simulink library "Driver_Long_Lat_Stanley"  (R2020b)
settings: Solver=VariableStepAuto  StartTime=0.0  StopTime=10.0  RelTol=1e-3
undefined symbols (not defined in the file): Driver
libraries: autolibutils x2, simulink x2, autolibsharedcommon x2, drivingvehiclecontroller x1, Maneuver_Get_Pose x1
(part 1 of 2)
Description:
  | Copyright 2020 The MathWorks, Inc.
settings Model: Creator=smiller  LastModifiedBy=smiller
settings DataIOCC: ReturnWorkspaceOutputs=off
settings DebuggingCC: ArithmeticOperatorsInVariantConditions=warning
settings SFSimCC: CustomCodeUndefinedFunction=UseInterfaceOnly

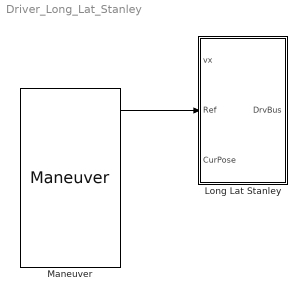
== system Driver_Long_Lat_Stanley ==
  Long Lat Stanley : Subsystem  mask{Driver=Driver}
  Maneuver : Maneuver_Get_Pose/Maneuver  Maneuver=Maneuver  popup_window=No
  wires:
  Maneuver/1 -> Long Lat Stanley/2(Ref)

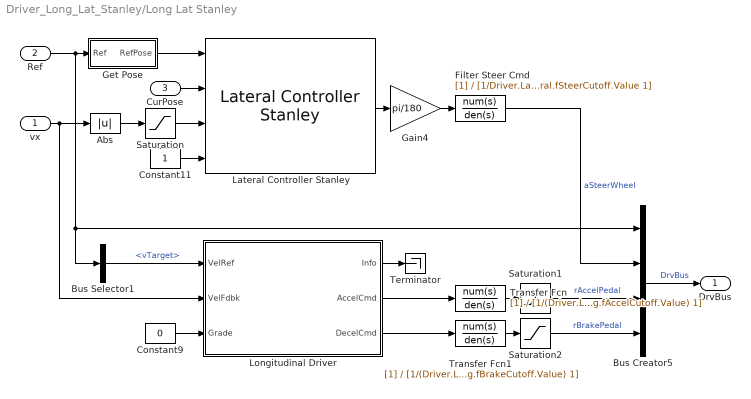
== system Driver_Long_Lat_Stanley/Long Lat Stanley ==
  vx : Inport
  Ref : Inport  Port=2
  CurPose : Inport  Port=3
  Abs : Abs
  Bus Creator5 : BusCreator  Inputs=4
  Bus Selector1 : BusSelector  OutputSignals=vTarget
  Constant11 : Constant
  Constant9 : Constant  Value=0
  Filter Steer Cmd : TransferFcn  Denominator=[1/Driver.Lateral.fSteerCutoff.Value 1]
  Gain4 : Gain  Gain=pi/180
  Get Pose : Subsystem
  Lateral Controller Stanley : drivingvehiclecontroller/Lateral Controller Stanley  ModelType=Kinematic bicycle model  PositionGainF=Driver.Lateral.NForward.Value  PositionGainR=Driver.Lateral.NReverse.Value  YawRateGain=0.2  DelayGain=0.2  VehicleMass=1575  Lf=1.2  Lr=1.6  TireStiffness=19000  Wheelbase=Driver.Lateral.xWheelbase.Value  MaxSteeringAngle=Driver.Lateral.aMaxSteer.Value
      settings: SourceProductName=Automated Driving System Toolbox
  Longitudinal Driver : Subsystem  SystemSampleTime=.01  mask(Longitudinal Driver){extAccelOvr=off, extDecelOvr=off, extAccelHld=off, extDecelHld=off, extAccelZero=off, extDecelZero=off, cntrlType=Predictive, shftType=None, velUnits=m/s, gearOut=off, Kp=15, Ki=1, Kff=.05, Kg=.01, VehVelVec=[0 100], KffVec=[.1 .1], KpVec=[10 10], KiVec=[5 5], KgVec=[0 0], m=Driver.Long.mVehicle.Value, Kpt=Driver.Long.FTractive.Value, tau=Driver.Long.tDriver.Value, L=Driver.Long.xPreview.Value, aR=Driver.Long.NDragRoll.Value, bR=Driver.Long.NDragRollDriveline.Value, cR=Driver.Long.NDragAero.Value, g=Driver.Long.gGravity.Value, vnom=100, Kaw=.1, tauerr=.03, tauPt=2, GearInit=0, tShift=.1, pdlVec=[0.1 0.4 0.5 0.9], upShftTbl=[-1 12.9375 26.4375 39.9375 51.18749999999999 62.4375 72.84375 83.25;-1 16.3125 29.8125 43.3125 54.5624 65.8125 76.78125 87.75;-1 19.6875 33.1875 46.68749999999999 57.9375 69.1875 80.71875 92.25;-1 33 52.5 77.25 100.5 138.75 161.875 185], dwnShftTbl=[1 9.5625 23.0625 36.5625 47.8125 59.0625 68.90625 78.75;1 12.9375 26.4375 39.9375 51.18749999999999 62.4375 72.84375 83.25;1 16.3125 29.8125 43.3125 54.562499 65.8125 76.78125 87.75;1 19.6875 33.1875 46.68749999999999 57.9375 69.1875 80.71875 92.25], tClutch=.5, tRev=.5, tPark=120, aMode=1, UpGearVec=[0  1  2  3  4  5  6  7], DownGearVec=[1  2  3  4  5  6  7  8]}
      mask prompts: extAccelOvr "autoblks_shared:autoblkLongitudinalDriver:blkPrm_extAccelOvr"; extDecelOvr "autoblks_shared:autoblkLongitudinalDriver:blkPrm_extDeccelOvr"; extAccelHld "autoblks_shared:autoblkLongitudinalDriver:blkPrm_extAccelHld"; extDecelHld "autoblks_shared:autoblkLongitudinalDriver:blkPrm_extDeccelHld"; extAccelZero "autoblks_shared:autoblkLongitudinalDriver:blkPrm_extAccelZero"; extDecelZero "autoblks_shared:autoblkLongitudinalDriver:blkPrm_extDeccelZero"; cntrlType "autoblks_shared:autoblkLongitudinalDriver:blkPrm_cntrlType"; shftType "autoblks_shared:autoblkLongitudinalDriver:blkPrm_shftType"; velUnits "autoblks_shared:autoblkLongitudinalDriver:blkPrm_velUnits"; gearOut "autoblks_shared:autoblkLongitudinalDriver:blkPrm_gearOut"; Kp "autoblks_shared:autoblkLongitudinalDriver:blkPrm_Kp"; Ki "autoblks_shared:autoblkLongitudinalDriver:blkPrm_Ki"; Kff "autoblks_shared:autoblkLongitudinalDriver:blkPrm_Kff"; Kg "autoblks_shared:autoblkLongitudinalDriver:blkPrm_Kg"; VehVelVec "autoblks_shared:autoblkLongitudinalDriver:blkPrm_VehVelVec"; KffVec "autoblks_shared:autoblkLongitudinalDriver:blkPrm_KffVec"; KpVec "autoblks_shared:autoblkLongitudinalDriver:blkPrm_KpVec"; KiVec "autoblks_shared:autoblkLongitudinalDriver:blkPrm_KiVec"; KgVec "autoblks_shared:autoblkLongitudinalDriver:blkPrm_KgVec"; m "autoblks_shared:autoblkLongitudinalDriver:blkPrm_m"; Kpt "autoblks_shared:autoblkLongitudinalDriver:blkPrm_Kpt"; tau "autoblks_shared:autoblkLongitudinalDriver:blkPrm_tau"; L "autoblks_shared:autoblkLongitudinalDriver:blkPrm_L"; aR "autoblks_shared:autoblkLongitudinalDriver:blkPrm_aR"; bR "autoblks_shared:autoblkLongitudinalDriver:blkPrm_bR"; cR "autoblks_shared:autoblkLongitudinalDriver:blkPrm_cR"; g "autoblks_shared:autoblkLongitudinalDriver:blkPrm_g"; vnom "autoblks_shared:autoblkLongitudinalDriver:blkPrm_vnom"; Kaw "autoblks_shared:autoblkLongitudinalDriver:blkPrm_Kaw"; tauerr "autoblks_shared:autoblkLongitudinalDriver:blkPrm_tauerr"; tauPt "autoblks_shared:autoblkLongitudinalDriver:blkPrm_tauPt"; GearInit "autoblks_shared:autoblkLongitudinalDriver:blkPrm_GearInit"; tShift "autoblks_shared:autoblkLongitudinalDriver:blkPrm_tShift"; pdlVec "autoblks_shared:autoblkLongitudinalDriver:blkPrm_pdlVec"; upShftTbl "autoblks_shared:autoblkLongitudinalDriver:blkPrm_upShftTbl"; dwnShftTbl "autoblks_shared:autoblkLongitudinalDriver:blkPrm_dwnShftTbl"; tClutch "autoblks_shared:autoblkLongitudinalDriver:blkPrm_tClutch"; tRev "autoblks_shared:autoblkLongitudinalDriver:blkPrm_tRev"; tPark "autoblks_shared:autoblkLongitudinalDriver:blkPrm_tPark"; UpGearVec "autoblks_shared:autoblkLongitudinalDriver:blkPrm_UpGearVec"; DownGearVec "autoblks_shared:autoblkLongitudinalDriver:blkPrm_DownGearVec"
      mask help: autoblks_shared:autoblkLongitudinalDriver:blkDesc
      mask init:
      | [~]=autosharedicon('autoliboperlong',gcb,0);
      mask Help: eval('autosharedhelp(''pbopmodlong'')');
      mask TypeOptions cntrlType: autoblks_shared:autoblkLongitudinalDriver:blkCmb_cntrlType_c1 | autoblks_shared:autoblkLongitudinalDriver:blkCmb_cntrlType_c2 | autoblks_shared:autoblkLongitudinalDriver:blkCmb_cntrlType_c3
      mask Callback cntrlType: [~]=autosharedicon('autoliboperlong',gcb,1);
      mask TypeOptions shftType: Longitudinal Driver/shftType
      mask Callback shftType: [~]=autosharedicon('autoliboperlong',gcb,1);
      mask TypeOptions velUnits: VelRef/Unit
      mask Callback velUnits: [~]=autosharedicon('autoliboperlong',gcb,1);
      mask DialogControl modeConfig Prompt: autoblks_shared:autoblkLongitudinalDriver:blkDlg_modeConfig
      mask DialogControl sigConfigPanel Prompt: autoblks_shared:autoblkLongitudinalDriver:blkDlg_sigConfigPanel
      mask DialogControl extAccelOvr Prompt: Accelerator override
      mask DialogControl extDecelOvr Prompt: Decelerator override
      mask DialogControl extAccelHld Prompt: Accelerator hold
      mask DialogControl extDecelHld Prompt: Decelerator hold
      mask DialogControl extAccelZero Prompt: Accelerator disable
      mask DialogControl extDecelZero Prompt: Decelerator disable
      mask DialogControl cntrlType Prompt: Control type, cntrlType:
      mask DialogControl shftType Prompt: Shift type, shftType:
      mask DialogControl velUnits Prompt: Reference and feedback units, velUnits [velUnits]:
      mask DialogControl gearOut Prompt: Output gear signal
      mask DialogControl CntrlParamPanel Prompt: autoblks_shared:autoblkLongitudinalDriver:blkDlg_CntrlParamPanel
      mask DialogControl PIParam Prompt: autoblks_shared:autoblkLongitudinalDriver:blkDlg_PIParam
      mask DialogControl Kp Prompt: Proportional gain, Kp []:
      mask DialogControl Ki Prompt: Integral gain, Ki []:
      mask DialogControl Kff Prompt: Velocity feed-forward, Kff []:
      mask DialogControl Kg Prompt: Grade angle feed-forward, Kg [1/deg]:
      mask DialogControl PISchedParam Prompt: autoblks_shared:autoblkLongitudinalDriver:blkDlg_PISchedParam
      mask DialogControl VehVelVec Prompt: Velocity gain breakpoints:
      mask DialogControl KffVec Prompt: Velocity feed-forward gain values, KffVec []:
      mask DialogControl KpVec Prompt: Proportional gain values, KpVec []:
      mask DialogControl KiVec Prompt: Integral gain values, KiVec []:
      mask DialogControl KgVec Prompt: Grade angle feed-forward values, KgVec [1/deg]:
      mask DialogControl PredParam Prompt: autoblks_shared:autoblkLongitudinalDriver:blkDlg_PredParam
      mask DialogControl m Prompt: Vehicle mass, m [kg]:
      mask DialogControl Kpt Prompt: Effective vehicle total tractive force, Kpt [N]:
      mask DialogControl tau Prompt: Driver response time, tau [s]:
      mask DialogControl L Prompt: Preview distance, L [m]:
      mask DialogControl aR Prompt: Rolling resistance coefficient, aR [N]:
      mask DialogControl bR Prompt: Rolling and driveline resistance coefficient, bR [N*s/m]:
      mask DialogControl cR Prompt: Aerodynamic drag coefficient, cR [N*s^2/m^2]:
      mask DialogControl g Prompt: Gravitational constant, g [m/s^2]:
      mask DialogControl vnom Prompt: Nominal speed, vnom [velUnits]:
      mask DialogControl Kaw Prompt: Anti-windup, Kaw []:
      mask DialogControl tauerr Prompt: Error filter time constant, tauerr [s]:
      mask DialogControl tauPt Prompt: Powertrain time constant, tauPt [s]:
      mask DialogControl shiftParamPanel Prompt: autoblks_shared:autoblkLongitudinalDriver:blkDlg_shiftParamPanel
      mask DialogControl GearInit Prompt: Initial gear, GearInit []:
      mask DialogControl tShift Prompt: Time required to shift, tShift [s]:
      mask DialogControl pdlVec Prompt: Up and down shift accelerator pedal positions, pdlVec []:
      mask DialogControl upShftTbl Prompt: Upshift velocity data table, upShftTbl [velUnits]:
      mask DialogControl dwnShftTbl Prompt: Downshift velocity data table, dwnShftTbl [velUnits]:
      mask DialogControl tClutch Prompt: Time required to shift, tClutch [s]:
      mask DialogControl tRev Prompt: Time required to engage reverse from neutral, tRev [s]:
      mask DialogControl tPark Prompt: Time required to engage park from neutral, tPark [s]:
      mask DialogControl UpGearVec Prompt: Upshift gear vector, UpGearVec []:
      mask DialogControl DownGearVec Prompt: Downshift gear vector, DownGearVec []:
      mask Display:
      | try
      |     IconInfo = autosharedicon('autoliboperlong', gcb, 4);
      | 
      |     image(IconInfo.image, IconInfo.position);
      | 
      |     for i = 1:numel(IconInfo.lconn)
      |         port_label('lconn', i, IconInfo.lconn{i})
      |     end
      | 
      |     for j = 1:numel(IconInfo.rconn)
      |         port_label('rconn', j, IconInfo.rconn{j})
      |     end
      | 
      |     for k = 1:numel(IconInfo.input)
      |         port_label('input', k, IconInfo.input{k})
      |     end
      | 
      |     for m = 1:numel(IconInfo.output)
      |         port_label('output', m, IconInfo.output{m})
      |     end
      | catch
      |     fprintf('Longitudinal \n Driver')
      | end
  Saturation : Saturate  UpperLimit=inf  LowerLimit=1e-9  ZeroCross=off
  Saturation1 : Saturate  UpperLimit=1  LowerLimit=0  ZeroCross=off
  Saturation2 : Saturate  UpperLimit=1  LowerLimit=0  ZeroCross=off
  Terminator : Terminator
  Transfer Fcn : TransferFcn  Denominator=[1/(Driver.Long.fAccelCutoff.Value) 1]
  Transfer Fcn1 : TransferFcn  Denominator=[1/(Driver.Long.fBrakeCutoff.Value) 1]
  DrvBus : Outport  VectorParamsAs1DForOutWhenUnconnected=off
  wires:
  Constant9/1 -> Longitudinal Driver/3(Grade)
  Bus Creator5/1 -> DrvBus/1  "DrvBus"
  Bus Selector1/1 -> Longitudinal Driver/1(VelRef)  "<vTarget>"
  Gain4/1 -> Filter Steer Cmd/1
  Lateral Controller Stanley/1 -> Gain4/1
  Longitudinal Driver/1(Info) -> Terminator/1
  Longitudinal Driver/2(AccelCmd) -> Transfer Fcn/1
  CurPose/1 -> Lateral Controller Stanley/2
  Longitudinal Driver/3(DecelCmd) -> Transfer Fcn1/1
  Abs/1 -> Saturation/1
  Transfer Fcn1/1 -> Saturation2/1
  Constant11/1 -> Lateral Controller Stanley/4
  Saturation2/1 -> Bus Creator5/4  "rBrakePedal"
  Saturation1/1 -> Bus Creator5/3  "rAccelPedal"
  Transfer Fcn/1 -> Saturation1/1
  vx/1 -> Longitudinal Driver/2(VelFdbk), Abs/1
  Ref/1 -> Bus Creator5/1, Bus Selector1/1, Get Pose/1(Ref)
  Get Pose/1(RefPose) -> Lateral Controller Stanley/1
  Filter Steer Cmd/1 -> Bus Creator5/2  "aSteerWheel"
  Saturation/1 -> Lateral Controller Stanley/3

== system Driver_Long_Lat_Stanley/Long Lat Stanley/Get Pose ==
  Ref : Inport
  Bus Selector : BusSelector  OutputSignals=x,y,ayaw
  Gain : Gain  Gain=180/pi
  Mux : Mux  Inputs=3
  RefPose : Outport  VectorParamsAs1DForOutWhenUnconnected=off
  wires:
  Bus Selector/1 -> Mux/1  "<x>"
  Ref/1 -> Bus Selector/1
  Mux/1 -> RefPose/1
  Bus Selector/2 -> Mux/2  "<y>"
  Bus Selector/3 -> Gain/1  "<ayaw>"
  Gain/1 -> Mux/3

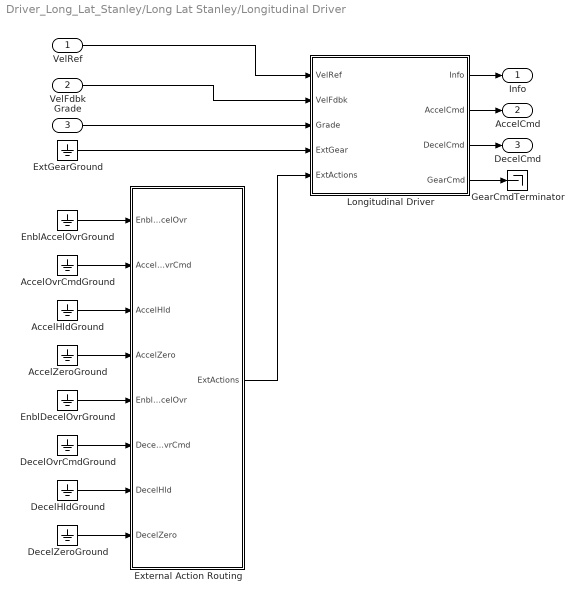
== system Driver_Long_Lat_Stanley/Long Lat Stanley/Longitudinal Driver ==
  VelRef : Inport  Unit=m/s
  VelFdbk : Inport  Port=2  Unit=m/s
  Grade : Inport  Port=3
  AccelHldGround : Ground
  AccelOvrCmdGround : Ground
  AccelZeroGround : Ground
  DecelHldGround : Ground
  DecelOvrCmdGround : Ground
  DecelZeroGround : Ground
  EnblAccelOvrGround : Ground
  EnblDecelOvrGround : Ground
  ExtGearGround : Ground
  External Action Routing : Subsystem
  GearCmdTerminator : Terminator
  Longitudinal Driver : Subsystem  mask(Longitudinal Driver Model){cntrlType=Predictive, shftType=None, vnom=vnom, Kp=Kp, Ki=Ki, Kaw=Kaw, Kff=Kff, Kg=Kg, tauerr=tauerr, tShift=tShift, tRev=tRev, tPark=tPark, pdlVec=pdlVec, upShftTbl=upShftTbl, dwnShftTbl=dwnShftTbl, GearInit=GearInit, tClutch=tClutch, VehVelVec=VehVelVec, KffVec=KffVec, KiVec=KiVec, KpVec=KpVec, KgVec=KgVec, m=m, Kpt=Kpt, Lvv=L, g=g, UpGearVec=UpGearVec, DownGearVec=DownGearVec, aMode=aMode, errUnit=m/s, aR=aR, bR=bR, cR=cR, tauPt=tauPt}
      mask prompts: cntrlType "Control type, cntrlType:"; shftType "Shift type, shftType:"; vnom "Nominal speed, vnom:"; Kp "Proportional gain, Kp:"; Ki "Integral gain, Ki:"; Kaw "Anti-windup, Kaw:"; Kff "Velocity feed-forward, Kff:"; Kg "Grade feed-forward, Kg:"; tauerr "Error filter time constant, tauerr [s]:"; tShift "Time required to shift. tShift [s]:"; tRev "Time required for reverse shift, tRev [s]:"; tPark "Time required to enter park, tPark [s]:"; pdlVec "Up and down shift accelerator pedal positions, pdlVec [-]:"; upShftTbl "Upshift speed data, upShftTbl []:"; dwnShftTbl "Downshift speed data, dwnShftTbl []:"; GearInit "Initial gear, GearInit [-]:"; tClutch "Time requried to shift, tClutch [s]:"; VehVelVec "Velocity gain breakpoints, VehVelVec []:"; KffVec "Velocity feed-forward gain values, KffVec []:Velocity feed-forward gain values, KffVec []:"; KiVec "Integral gain values, KiVec []:"; KpVec "Proportional gain values, KpVec []:"; KgVec "Grade feed-forward values, KgVec []:Grade feed-forward values, KgVec []:Grade feed-forward values, KgVec []:Grade feed-forward values, KgVec []:Grade feed-forward values, KgVec []:"; m "Vehicle mass, m [m]:"; Kpt "Tractive force, Kpt [N]:"; Lvv "Preview distance, Lvv [m]:"; g "Gravitational constant, g, [m/s^2]:"; errUnit "Error units, errUnit"; aR "Static resistance, aR [N]:"; bR "Linear resistance, bR [N*s/m]:"; cR "Quadratic resistance, cR [N*s^2/m^2]:"; tauPt "Powertrain time constant, tauPt [s]:"
      mask help: A parametric longitudinal speed tracking controller for generating normalized acceleration and braking commands based on reference and feedback velocities.
      mask init:
      | [~]=autosharedicon('autoliboperlong',gcb,1);
      mask Help: eval('autoblkshelp(''pbopmodlong'')');
      mask TypeOptions cntrlType: PI | Scheduled PI | Predictive
      mask TypeOptions shftType: None | Reverse, Neutral, Drive | Scheduled | External
      mask TypeOptions errUnit: Routing/error signal spec/Unit
  Info : Outport  InitialOutput=0  VectorParamsAs1DForOutWhenUnconnected=off
  AccelCmd : Outport  Port=2  VectorParamsAs1DForOutWhenUnconnected=off
  DecelCmd : Outport  Port=3  VectorParamsAs1DForOutWhenUnconnected=off
  wires:
  ExtGearGround/1 -> Longitudinal Driver/4(ExtGear)
  Longitudinal Driver/4(GearCmd) -> GearCmdTerminator/1
  EnblDecelOvrGround/1 -> External Action Routing/5(EnblDecelOvr)
  AccelZeroGround/1 -> External Action Routing/4(AccelZero)
  DecelZeroGround/1 -> External Action Routing/8(DecelZero)
  DecelOvrCmdGround/1 -> External Action Routing/6(DecelOvrCmd)
  DecelHldGround/1 -> External Action Routing/7(DecelHld)
  AccelHldGround/1 -> External Action Routing/3(AccelHld)
  EnblAccelOvrGround/1 -> External Action Routing/1(EnblAccelOvr)
  AccelOvrCmdGround/1 -> External Action Routing/2(AccelOvrCmd)
  External Action Routing/1(ExtActions) -> Longitudinal Driver/5(ExtActions)
  Grade/1 -> Longitudinal Driver/3(Grade)
  Longitudinal Driver/3(DecelCmd) -> DecelCmd/1
  Longitudinal Driver/2(AccelCmd) -> AccelCmd/1
  Longitudinal Driver/1(Info) -> Info/1
  VelFdbk/1 -> Longitudinal Driver/2(VelFdbk)
  VelRef/1 -> Longitudinal Driver/1(VelRef)

== system Driver_Long_Lat_Stanley/Long Lat Stanley/Longitudinal Driver/External Action Routing ==
  EnblAccelOvr : Inport  OutDataTypeStr=boolean  Unit=1
  AccelOvrCmd : Inport  Port=2  OutDataTypeStr=double  Unit=1
  AccelHld : Inport  Port=3  OutDataTypeStr=boolean  Unit=1
  AccelZero : Inport  Port=4  OutDataTypeStr=boolean  Unit=1
  EnblDecelOvr : Inport  Port=5  OutDataTypeStr=boolean  Unit=1
  DecelOvrCmd : Inport  Port=6  OutDataTypeStr=double  Unit=1
  DecelHld : Inport  Port=7  OutDataTypeStr=boolean  Unit=1
  DecelZero : Inport  Port=8  OutDataTypeStr=boolean  Unit=1
  Bus Creator2 : BusCreator  Inputs=8
  ExtActions : Outport
  wires:
  Bus Creator2/1 -> ExtActions/1  "ExtActions"
  DecelZero/1 -> Bus Creator2/8  "DecelZero"
  DecelHld/1 -> Bus Creator2/7  "DecelHld"
  DecelOvrCmd/1 -> Bus Creator2/6  "DecelOvrCmd"
  EnblDecelOvr/1 -> Bus Creator2/5  "EnblDecelOvr"
  AccelZero/1 -> Bus Creator2/4  "AccelZero"
  AccelHld/1 -> Bus Creator2/3  "AccelHld"
  AccelOvrCmd/1 -> Bus Creator2/2  "AccelOvrCmd"
  EnblAccelOvr/1 -> Bus Creator2/1  "EnblAccelOvr"

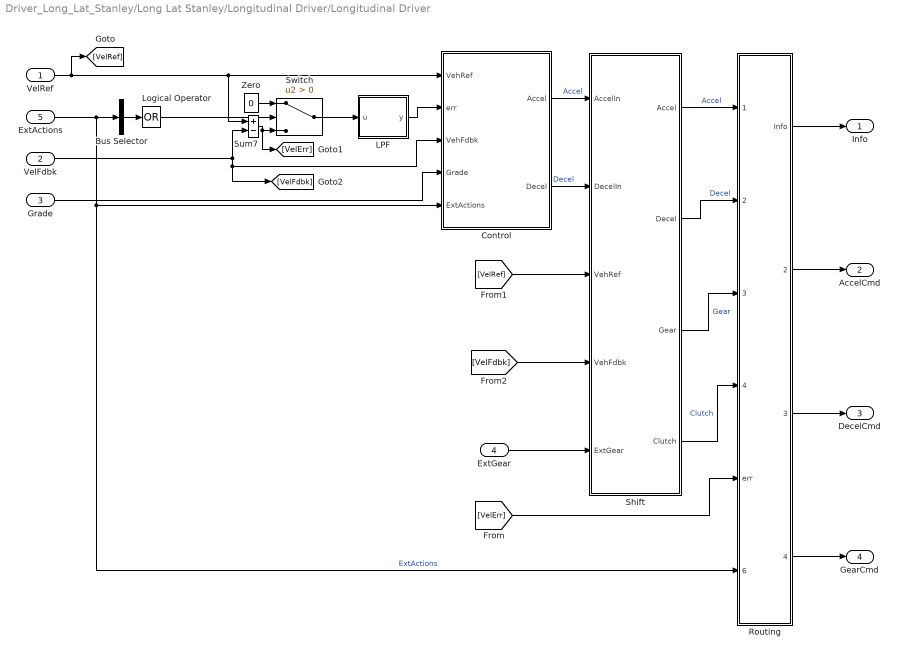
== system Driver_Long_Lat_Stanley/Long Lat Stanley/Longitudinal Driver/Longitudinal Driver ==
  VelRef : Inport
  VelFdbk : Inport  Port=2
  Grade : Inport  Port=3  Unit=deg
  ExtGear : Inport  Port=4  Unit=1
  ExtActions : Inport  Port=5
  Bus Selector : BusSelector  OutputSignals=EnblAccelOvr,AccelHld,AccelZero,EnblDecelOvr,DecelZero,DecelHld  OutputAsBus=on
  Control : Subsystem  Variant=on  VariantControlMode=label  LabelModeActiveChoice=2
  LPF : Subsystem  Variant=on  VariantControlMode=label  LabelModeActiveChoice=0
  Logical Operator : Logic  Operator=OR  Inputs=1  AllPortsSameDT=off  OutDataTypeStr=boolean
  Routing : Subsystem
  Shift : Subsystem  Variant=on  VariantControlMode=label  LabelModeActiveChoice=0
  Sum7 : Sum  Inputs=+-  InputSameDT=on  SaturateOnIntegerOverflow=on  OutDataTypeStr=Inherit: Same as first input
  Switch : Switch  Criteria=u2 > Threshold
  Zero : Constant  Value=0  OutDataTypeStr=Inherit: Inherit via back propagation
  Info : Outport  InitialOutput=0  VectorParamsAs1DForOutWhenUnconnected=off
  AccelCmd : Outport  Port=2  Unit=one  InitialOutput=0  VectorParamsAs1DForOutWhenUnconnected=off
  DecelCmd : Outport  Port=3  Unit=one  InitialOutput=0  VectorParamsAs1DForOutWhenUnconnected=off
  GearCmd : Outport  Port=4  Unit=one  InitialOutput=0  VectorParamsAs1DForOutWhenUnconnected=off
  wires:
  Control/1(Accel) -> Shift/1(AccelIn)  "Accel"
  [VelFdbk] -> Shift/4(VehFdbk)
  Control/2(Decel) -> Shift/2(DecelIn)  "Decel"
  Routing/3(DecelCmd) -> DecelCmd/1
  [VelErr] -> Routing/5(err)
  [VelRef] -> Shift/3(VehRef)
  Routing/4(GearCmd) -> GearCmd/1
  Shift/3(Gear) -> Routing/3(GearIn)  "Gear"
  Routing/1(Info) -> Info/1
  Shift/2(Decel) -> Routing/2(DecelIn)  "Decel"
  Shift/4(Clutch) -> Routing/4(Clutch)  "Clutch"
  Routing/2(AccelCmd) -> AccelCmd/1
  Grade/1 -> Control/4(Grade)
  Sum7/1 -> Switch/3, [VelErr]
  Shift/1(Accel) -> Routing/1(AccelIn)  "Accel"
  LPF/1(y) -> Control/2(err)
  ExtGear/1 -> Shift/5(ExtGear)
  VelRef/1 -> Control/1(VehRef), Sum7/1, [VelRef]
  VelFdbk/1 -> [VelFdbk], Control/3(VehFdbk), Sum7/2
  ExtActions/1 -> Routing/6(ExtActions), Control/5(ExtActions), Bus Selector/1  "ExtActions"
  Switch/1 -> LPF/1(u)
  Logical Operator/1 -> Switch/2
  Zero/1 -> Switch/1
  Bus Selector/1 -> Logical Operator/1

== system Driver_Long_Lat_Stanley/Long Lat Stanley/Longitudinal Driver/Longitudinal Driver/Control ==
  note: 1) Add Subsystem or Model blocks as valid variant choices.
      | 2) You cannot connect blocks at this level. At simulation, connectivity is automatically
      | determined, based on the active variant and port name matching.
  VehRef : Inport
  err : Inport  Port=2
  VehFdbk : Inport  Port=3
  Grade : Inport  Port=4
  ExtActions : Inport  Port=5
  Mapped : Subsystem  VariantControl=1
  Predictive : Subsystem  VariantControl=2
  Scalar : Subsystem  VariantControl=0
  Accel : Outport  VectorParamsAs1DForOutWhenUnconnected=off
  Decel : Outport  Port=2  VectorParamsAs1DForOutWhenUnconnected=off

== system Driver_Long_Lat_Stanley/Long Lat Stanley/Longitudinal Driver/Longitudinal Driver/LPF ==
  note: 1) Add Subsystem or Model blocks as valid variant choices.
      | 2) You cannot connect blocks at this level. At simulation, connectivity is automatically
      | determined, based on the active variant and port name matching.
  u : Inport
  LPF : Subsystem  VariantControl=1
  pass : Subsystem  VariantControl=0
  y : Outport  VectorParamsAs1DForOutWhenUnconnected=off

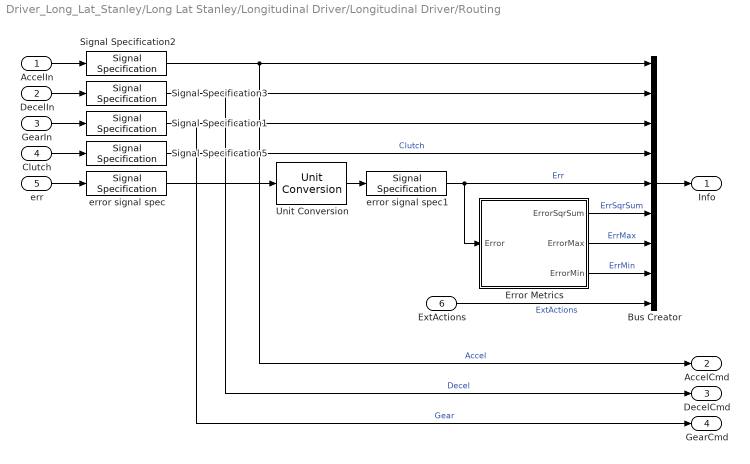
== system Driver_Long_Lat_Stanley/Long Lat Stanley/Longitudinal Driver/Longitudinal Driver/Routing ==
  AccelIn : Inport
  DecelIn : Inport  Port=2
  GearIn : Inport  Port=3
  Clutch : Inport  Port=4
  err : Inport  Port=5
  ExtActions : Inport  Port=6
  Bus Creator : BusCreator  Inputs=9
  Error Metrics : Subsystem
  Signal Specification{1..3,5} (4 alike) : SignalSpecification  Unit=1
  Unit Conversion : UnitConversion
  error signal spec : SignalSpecification  Unit=m/s
  error signal spec1 : SignalSpecification  Unit=m/s
  Info : Outport  VectorParamsAs1DForOutWhenUnconnected=off
  AccelCmd : Outport  Port=2  VectorParamsAs1DForOutWhenUnconnected=off
  DecelCmd : Outport  Port=3  VectorParamsAs1DForOutWhenUnconnected=off
  GearCmd : Outport  Port=4  VectorParamsAs1DForOutWhenUnconnected=off
  wires:
  GearIn/1 -> Signal Specification1/1
  Signal Specification2/1 -> AccelCmd/1, Bus Creator/1  "Accel"
  error signal spec/1 -> Unit Conversion/1
  Error Metrics/1(ErrorSqrSum) -> Bus Creator/6  "ErrSqrSum"
  Error Metrics/3(ErrorMin) -> Bus Creator/8  "ErrMin"
  Signal Specification5/1 -> Bus Creator/4  "Clutch"
  Signal Specification3/1 -> DecelCmd/1, Bus Creator/2  "Decel"
  Signal Specification1/1 -> GearCmd/1, Bus Creator/3  "Gear"
  AccelIn/1 -> Signal Specification2/1
  Error Metrics/2(ErrorMax) -> Bus Creator/7  "ErrMax"
  Bus Creator/1 -> Info/1
  Clutch/1 -> Signal Specification5/1
  DecelIn/1 -> Signal Specification3/1
  err/1 -> error signal spec/1
  error signal spec1/1 -> Error Metrics/1(Error), Bus Creator/5  "Err"
  Unit Conversion/1 -> error signal spec1/1
  ExtActions/1 -> Bus Creator/9  "ExtActions"

== system Driver_Long_Lat_Stanley/Long Lat Stanley/Longitudinal Driver/Longitudinal Driver/Shift ==
  note: 1) Add Subsystem or Model blocks as valid variant choices.
      | 2) You cannot connect blocks at this level. At simulation, connectivity is automatically
      | determined, based on the active variant and port name matching.
  AccelIn : Inport
  DecelIn : Inport  Port=2
  VehRef : Inport  Port=3
  VehFdbk : Inport  Port=4
  ExtGear : Inport  Port=5
  Basic : Subsystem  VariantControl=1
  External : Subsystem  VariantControl=4
  None : Subsystem  VariantControl=0
  Scheduled : Subsystem  VariantControl=3
  Accel : Outport  VectorParamsAs1DForOutWhenUnconnected=off
  Decel : Outport  Port=2  VectorParamsAs1DForOutWhenUnconnected=off
  Gear : Outport  Port=3  VectorParamsAs1DForOutWhenUnconnected=off
  Clutch : Outport  Port=4  VectorParamsAs1DForOutWhenUnconnected=off

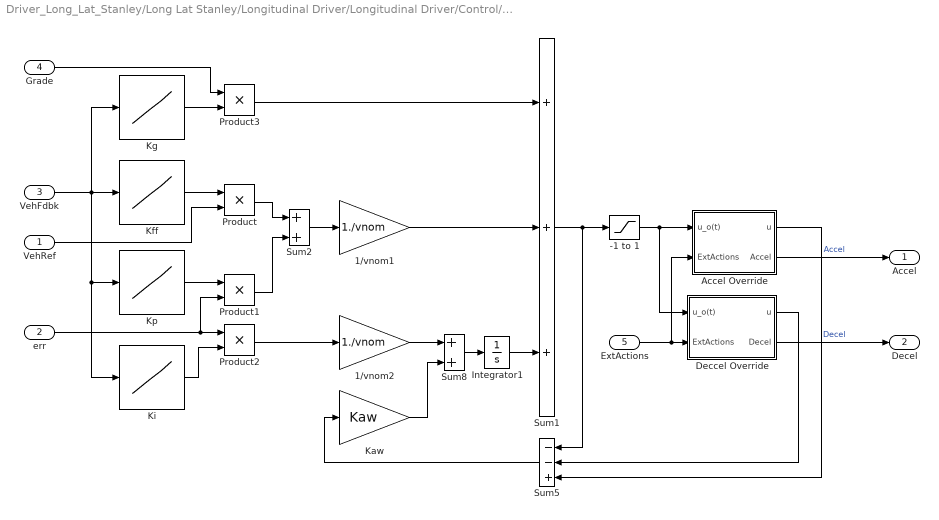
== system Driver_Long_Lat_Stanley/Long Lat Stanley/Longitudinal Driver/Longitudinal Driver/Control/Mapped ==
  VehRef : Inport
  err : Inport  Port=2
  VehFdbk : Inport  Port=3
  Grade : Inport  Port=4  Unit=deg
  ExtActions : Inport  Port=5
  "-1 to 1 " : Saturate  UpperLimit=1  LowerLimit=-1
  1/vnom1 : Gain  Gain=1./vnom  SaturateOnIntegerOverflow=on  OutDataTypeStr=Inherit: Same as input  ParamDataTypeStr=Inherit: Same as input
  1/vnom2 : Gain  Gain=1./vnom  SaturateOnIntegerOverflow=on  OutDataTypeStr=Inherit: Same as input  ParamDataTypeStr=Inherit: Same as input
  Accel Override : Subsystem
  Deccel Override : Subsystem
  Integrator1 : Integrator  LimitOutput=on  UpperSaturationLimit=1  LowerSaturationLimit=-1
  Kaw : Gain  Gain=Kaw  SaturateOnIntegerOverflow=on  OutDataTypeStr=Inherit: Same as input  ParamDataTypeStr=Inherit: Same as input
  Kff : Lookup_n-D  NumberOfTableDimensions=1  BreakpointsForDimension1=VehVelVec  Table=KffVec  InternalRulePriority=Speed  RndMeth=Simplest  InputSameDT=on
  Kg : Lookup_n-D  NumberOfTableDimensions=1  BreakpointsForDimension1=VehVelVec  Table=KgVec  InternalRulePriority=Speed  RndMeth=Simplest  InputSameDT=on
  Ki : Lookup_n-D  NumberOfTableDimensions=1  BreakpointsForDimension1=VehVelVec  Table=KiVec  InternalRulePriority=Speed  RndMeth=Simplest  InputSameDT=on
  Kp : Lookup_n-D  NumberOfTableDimensions=1  BreakpointsForDimension1=VehVelVec  Table=KpVec  InternalRulePriority=Speed  RndMeth=Simplest  InputSameDT=on
  Product{,1..3} (4 alike) : Product
  Sum1 : Sum  Inputs=+++  InputSameDT=on  SaturateOnIntegerOverflow=on  OutDataTypeStr=Inherit: Same as first input
  Sum2 : Sum  InputSameDT=on  SaturateOnIntegerOverflow=on  OutDataTypeStr=Inherit: Same as first input
  Sum5 : Sum  Inputs=--+  InputSameDT=on  SaturateOnIntegerOverflow=on  OutDataTypeStr=Inherit: Same as first input
  Sum8 : Sum  InputSameDT=on  SaturateOnIntegerOverflow=on  OutDataTypeStr=Inherit: Same as first input
  Accel : Outport  Unit=one  InitialOutput=0  VectorParamsAs1DForOutWhenUnconnected=off
  Decel : Outport  Port=2  Unit=one  InitialOutput=0  VectorParamsAs1DForOutWhenUnconnected=off
  wires:
  Deccel Override/2(Decel) -> Decel/1  "Decel"
  "-1 to 1 "/1 -> Deccel Override/1(u_o(t)), Accel Override/1(u_o(t))
  Sum8/1 -> Integrator1/1
  Product3/1 -> Sum1/1
  Kaw/1 -> Sum8/2
  1/vnom2/1 -> Sum8/1
  1/vnom1/1 -> Sum1/2
  Sum1/1 -> Sum5/1, "-1 to 1 "/1
  Sum5/1 -> Kaw/1
  Integrator1/1 -> Sum1/3
  err/1 -> Product1/2, Product2/1
  Grade/1 -> Product3/1
  Product/1 -> Sum2/1
  Kff/1 -> Product/1
  Kp/1 -> Product1/1
  Product1/1 -> Sum2/2
  VehFdbk/1 -> Ki/1, Kp/1, Kg/1, Kff/1
  Ki/1 -> Product2/2
  Product2/1 -> 1/vnom2/1
  Kg/1 -> Product3/2
  Sum2/1 -> 1/vnom1/1
  VehRef/1 -> Product/2
  ExtActions/1 -> Deccel Override/2(ExtActions), Accel Override/2(ExtActions)
  Accel Override/2(Accel) -> Accel/1  "Accel"
  Deccel Override/1(u) -> Sum5/2
  Accel Override/1(u) -> Sum5/3

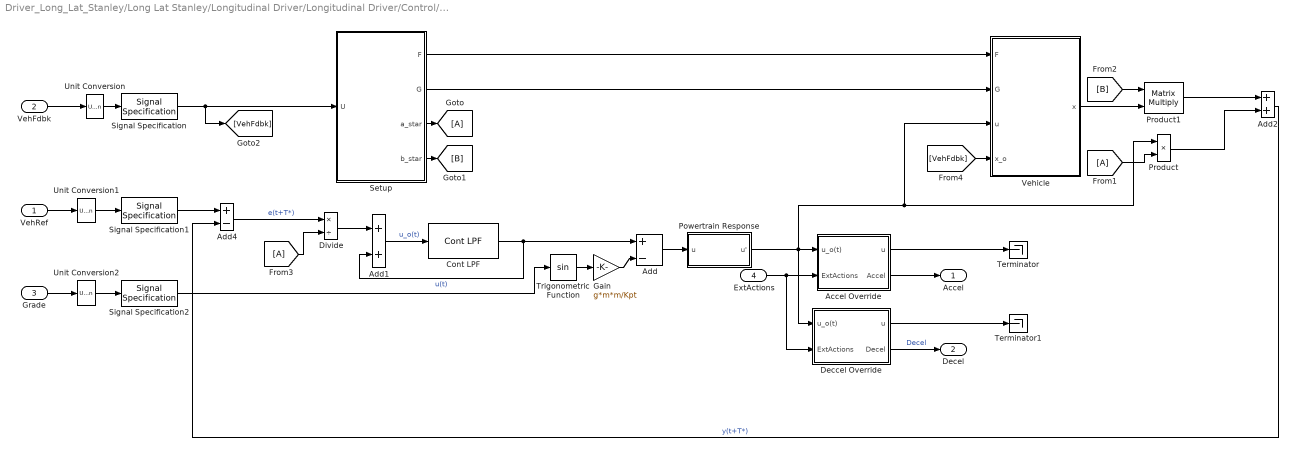
== system Driver_Long_Lat_Stanley/Long Lat Stanley/Longitudinal Driver/Longitudinal Driver/Control/Predictive ==
  VehRef : Inport
  VehFdbk : Inport  Port=2
  Grade : Inport  Port=3
  ExtActions : Inport  Port=4
  Accel Override : Subsystem
  Add : Sum  Inputs=+-
  Add1 : Sum
  Add2 : Sum
  Add4 : Sum  Inputs=+-
  Cont LPF : autolibutils/Cont LPF  wc=(1/tau)*pi*2  aMode=aMode
      settings: SourceProductBaseCode=PW,MT,UV,VE,VP
  Deccel Override : Subsystem
  Divide : Product  Inputs=*/
  Gain : Gain  Gain=g*m*m/Kpt
  Powertrain Response : Subsystem  Variant=on  VariantControlMode=label  VariantControl=Variant1  LabelModeActiveChoice=0
  Product : Product
  Product1 : Product  Multiplication=Matrix(*)
  Setup : MATLAB Function  TreatAsAtomicUnit=on
  Signal Specification : SignalSpecification  Unit=m/s
  Signal Specification1 : SignalSpecification  Unit=m/s
  Signal Specification2 : SignalSpecification  Unit=rad
  Terminator : Terminator
  Terminator1 : Terminator
  Trigonometric Function : Trigonometry
  Unit Conversion : UnitConversion
  Unit Conversion1 : UnitConversion
  Unit Conversion2 : UnitConversion
  Vehicle : MATLAB Function  TreatAsAtomicUnit=on
  Accel : Outport  VectorParamsAs1DForOutWhenUnconnected=off
  Decel : Outport  Port=2  VectorParamsAs1DForOutWhenUnconnected=off
  wires:
  Add1/1 -> Cont LPF/1  "u_o(t)"
  Cont LPF/1 -> Add/1, Add1/2  "u(t)"
  Signal Specification2/1 -> Trigonometric Function/1
  Gain/1 -> Add/2
  Add4/1 -> Divide/1  "e(t+T*)"
  Deccel Override/2(Decel) -> Decel/1  "Decel"
  [B] -> Product1/1
  Vehicle/1(x) -> Product1/2
  Add2/1 -> Add4/2  "y(t+T*)"
  Signal Specification1/1 -> Add4/1
  Product1/1 -> Add2/1
  [A] -> Divide/2
  Signal Specification/1 -> [VehFdbk], Setup/1(U)
  Product/1 -> Add2/2
  Setup/1(F) -> Vehicle/1(F)
  Setup/3(a_star) -> [A]
  Divide/1 -> Add1/1
  Setup/4(b_star) -> [B]
  [A] -> Product/2
  [VehFdbk] -> Vehicle/4(x_o)
  Trigonometric Function/1 -> Gain/1
  Unit Conversion1/1 -> Signal Specification1/1
  Unit Conversion/1 -> Signal Specification/1
  VehFdbk/1 -> Unit Conversion/1
  VehRef/1 -> Unit Conversion1/1
  Unit Conversion2/1 -> Signal Specification2/1
  Grade/1 -> Unit Conversion2/1
  Setup/2(G) -> Vehicle/2(G)
  Add/1 -> Powertrain Response/1("u ")
  Accel Override/2(Accel) -> Accel/1
  ExtActions/1 -> Deccel Override/2(ExtActions), Accel Override/2(ExtActions)
  Accel Override/1(u) -> Terminator/1
  Powertrain Response/1(" u'") -> Deccel Override/1(u_o(t)), Accel Override/1(u_o(t)), Product/1, Vehicle/3(u)
  Deccel Override/1(u) -> Terminator1/1

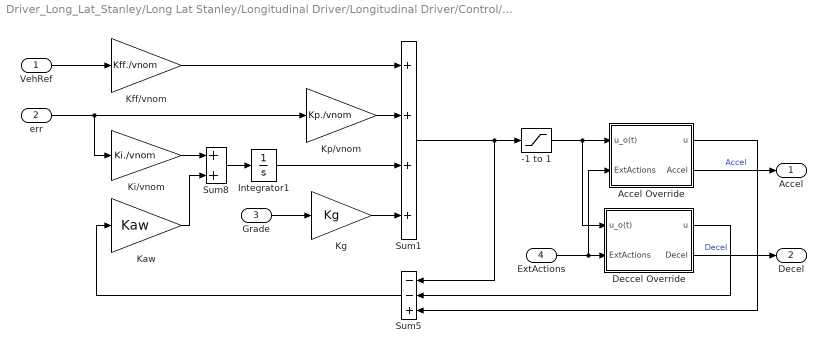
== system Driver_Long_Lat_Stanley/Long Lat Stanley/Longitudinal Driver/Longitudinal Driver/Control/Scalar ==
  VehRef : Inport
  err : Inport  Port=2
  Grade : Inport  Port=3  Unit=deg
  ExtActions : Inport  Port=4
  "-1 to 1 " : Saturate  UpperLimit=1  LowerLimit=-1
  Accel Override : Subsystem
  Deccel Override : Subsystem
  Integrator1 : Integrator  LimitOutput=on  UpperSaturationLimit=1  LowerSaturationLimit=-1
  Kaw : Gain  Gain=Kaw  SaturateOnIntegerOverflow=on  OutDataTypeStr=Inherit: Same as input  ParamDataTypeStr=Inherit: Same as input
  Kff/vnom : Gain  Gain=Kff./vnom  SaturateOnIntegerOverflow=on  OutDataTypeStr=Inherit: Same as input  ParamDataTypeStr=Inherit: Same as input
  Kg : Gain  Gain=Kg  SaturateOnIntegerOverflow=on  OutDataTypeStr=Inherit: Same as input  ParamDataTypeStr=Inherit: Same as input
  Ki/vnom : Gain  Gain=Ki./vnom  SaturateOnIntegerOverflow=on  OutDataTypeStr=Inherit: Same as input  ParamDataTypeStr=Inherit: Same as input
  Kp/vnom : Gain  Gain=Kp./vnom  SaturateOnIntegerOverflow=on  OutDataTypeStr=Inherit: Same as input  ParamDataTypeStr=Inherit: Same as input
  Sum1 : Sum  Inputs=++++  InputSameDT=on  SaturateOnIntegerOverflow=on  OutDataTypeStr=Inherit: Same as first input
  Sum5 : Sum  Inputs=--+  InputSameDT=on  SaturateOnIntegerOverflow=on  OutDataTypeStr=Inherit: Same as first input
  Sum8 : Sum  InputSameDT=on  SaturateOnIntegerOverflow=on  OutDataTypeStr=Inherit: Same as first input
  Accel : Outport  Unit=one  InitialOutput=0  VectorParamsAs1DForOutWhenUnconnected=off
  Decel : Outport  Port=2  Unit=one  InitialOutput=0  VectorParamsAs1DForOutWhenUnconnected=off
  wires:
  Grade/1 -> Kg/1
  err/1 -> Ki/vnom/1, Kp/vnom/1
  Accel Override/2(Accel) -> Accel/1  "Accel"
  Integrator1/1 -> Sum1/3
  Sum5/1 -> Kaw/1
  VehRef/1 -> Kff/vnom/1
  Sum1/1 -> "-1 to 1 "/1, Sum5/1
  Kp/vnom/1 -> Sum1/2
  Ki/vnom/1 -> Sum8/1
  Kaw/1 -> Sum8/2
  Kg/1 -> Sum1/4
  Sum8/1 -> Integrator1/1
  Kff/vnom/1 -> Sum1/1
  "-1 to 1 "/1 -> Deccel Override/1(u_o(t)), Accel Override/1(u_o(t))
  Deccel Override/2(Decel) -> Decel/1  "Decel"
  ExtActions/1 -> Accel Override/2(ExtActions), Deccel Override/2(ExtActions)
  Deccel Override/1(u) -> Sum5/2
  Accel Override/1(u) -> Sum5/3

== system Driver_Long_Lat_Stanley/Long Lat Stanley/Longitudinal Driver/Longitudinal Driver/LPF/LPF ==
  u : Inport
  Constant : Constant  Value=tauerr  SampleTime=-1
  Divide : Product  Inputs=/
  Error LPF : autolibutils/Cont LPF Dyn  aMode=aMode  dataType=off
      settings: SourceProductBaseCode=PW,MT,UV,VE,VP
  y : Outport  VectorParamsAs1DForOutWhenUnconnected=off
  wires:
  u/1 -> Error LPF/1
  Error LPF/1 -> y/1
  Divide/1 -> Error LPF/2
  Constant/1 -> Divide/1

== system Driver_Long_Lat_Stanley/Long Lat Stanley/Longitudinal Driver/Longitudinal Driver/LPF/pass ==
  u : Inport
  y : Outport  VectorParamsAs1DForOutWhenUnconnected=off
  wires:
  u/1 -> y/1

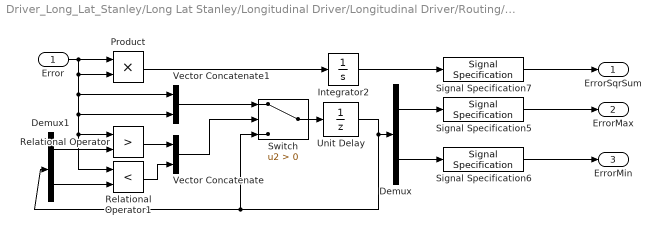
== system Driver_Long_Lat_Stanley/Long Lat Stanley/Longitudinal Driver/Longitudinal Driver/Routing/Error Metrics ==
  Error : Inport
  Demux : Demux  Outputs=2
  Demux1 : Demux  Outputs=2
  Integrator2 : Integrator  UpperSaturationLimit=1  LowerSaturationLimit=-1  ZeroCross=off
  Product : Product
  Relational Operator : RelationalOperator  Operator=>  OutDataTypeStr=boolean  ZeroCross=off  RndMeth=Simplest
  Relational Operator1 : RelationalOperator  Operator=<  OutDataTypeStr=boolean  ZeroCross=off  RndMeth=Simplest
  Signal Specification5 : SignalSpecification  Unit=m/s
  Signal Specification6 : SignalSpecification  Unit=m/s
  Signal Specification7 : SignalSpecification  Unit=m^2/s^2
  Switch : Switch  Criteria=u2 > Threshold
  Unit Delay : UnitDelay  InitialCondition=[0,0]  SampleTime=-1  HasFrameUpgradeWarning=on
  Vector Concatenate : Concatenate
  Vector Concatenate1 : Concatenate
  ErrorSqrSum : Outport  VectorParamsAs1DForOutWhenUnconnected=off
  ErrorMax : Outport  Port=2  VectorParamsAs1DForOutWhenUnconnected=off
  ErrorMin : Outport  Port=3  VectorParamsAs1DForOutWhenUnconnected=off
  wires:
  Integrator2/1 -> Signal Specification7/1
  Product/1 -> Integrator2/1
  Error/1 -> Product/2, Vector Concatenate1/2, Relational Operator1/1, Relational Operator/1, Vector Concatenate1/1, Product/1
  Switch/1 -> Unit Delay/1
  Unit Delay/1 -> Switch/3, Demux1/1, Demux/1
  Relational Operator1/1 -> Vector Concatenate/2
  Relational Operator/1 -> Vector Concatenate/1
  Vector Concatenate1/1 -> Switch/1
  Demux/1 -> Signal Specification5/1
  Demux/2 -> Signal Specification6/1
  Demux1/2 -> Relational Operator1/2
  Demux1/1 -> Relational Operator/2
  Vector Concatenate/1 -> Switch/2
  Signal Specification7/1 -> ErrorSqrSum/1
  Signal Specification6/1 -> ErrorMin/1
  Signal Specification5/1 -> ErrorMax/1

== system Driver_Long_Lat_Stanley/Long Lat Stanley/Longitudinal Driver/Longitudinal Driver/Shift/Basic ==
  AccelIn : Inport
  DecelIn : Inport  Port=2
  VehRef : Inport  Port=3
  VehFdbk : Inport  Port=4
  ExtGear : Inport  Port=5
  Constant1 : Constant  Value=0
  Reverse Change : Subsystem
  Shift Controller : Stateflow chart  TreatAsAtomicUnit=on
  Terminator : Terminator
  Accel : Outport  VectorParamsAs1DForOutWhenUnconnected=off
  Decel : Outport  Port=2  VectorParamsAs1DForOutWhenUnconnected=off
  Gear : Outport  Port=3  VectorParamsAs1DForOutWhenUnconnected=off
  Clutch : Outport  Port=4  VectorParamsAs1DForOutWhenUnconnected=off
  wires:
  Shift Controller/1(Gear) -> Gear/1, Reverse Change/3(GearIn)
  AccelIn/1 -> Shift Controller/1(pedal), Reverse Change/1(AccelIn)
  VehRef/1 -> [VehRef], Shift Controller/3(VehRef)
  DecelIn/1 -> Shift Controller/2(Brake), Reverse Change/2(DecelIn)
  Reverse Change/1(Accel) -> Accel/1
  Reverse Change/2(Decel) -> Decel/1
  Constant1/1 -> Clutch/1
  ExtGear/1 -> Terminator/1
  [VehRef] -> Reverse Change/4(VehRef)
  VehFdbk/1 -> Shift Controller/4(speed)

== system Driver_Long_Lat_Stanley/Long Lat Stanley/Longitudinal Driver/Longitudinal Driver/Shift/External ==
  AccelIn : Inport
  DecelIn : Inport  Port=2
  VehRef : Inport  Port=3
  VehFdbk : Inport  Port=4
  ExtGear : Inport  Port=5
  Constant1 : Constant  Value=0
  Reverse Change : autolibsharedcommon/Longitudinal Driver/Shift/Basic/Reverse Change  SystemSampleTime=-1  VariantActivationTime=update diagram  Latency=0  AutoFrameSizeCalculation=off
      settings: SourceProductBaseCode=PW,MT,UV,VE,VP
  Terminator1 : Terminator
  Accel : Outport  VectorParamsAs1DForOutWhenUnconnected=off
  Decel : Outport  Port=2  VectorParamsAs1DForOutWhenUnconnected=off
  Gear : Outport  Port=3  VectorParamsAs1DForOutWhenUnconnected=off
  Clutch : Outport  Port=4  VectorParamsAs1DForOutWhenUnconnected=off
  wires:
  ExtGear/1 -> Gear/1, Reverse Change/3
  AccelIn/1 -> Reverse Change/1
  DecelIn/1 -> Reverse Change/2
  Reverse Change/2 -> Decel/1
  Reverse Change/1 -> Accel/1
  Constant1/1 -> Clutch/1
  VehRef/1 -> Reverse Change/4
  VehFdbk/1 -> Terminator1/1

== system Driver_Long_Lat_Stanley/Long Lat Stanley/Longitudinal Driver/Longitudinal Driver/Shift/None ==
  AccelIn : Inport
  DecelIn : Inport  Port=2
  VehRef : Inport  Port=3
  VehFdbk : Inport  Port=4
  ExtGear : Inport  Port=5
  Constant : Constant
  Constant1 : Constant  Value=0
  Terminator1 : Terminator
  Terminator2 : Terminator
  Terminator3 : Terminator
  Accel : Outport  VectorParamsAs1DForOutWhenUnconnected=off
  Decel : Outport  Port=2  VectorParamsAs1DForOutWhenUnconnected=off
  Gear : Outport  Port=3  VectorParamsAs1DForOutWhenUnconnected=off
  Clutch : Outport  Port=4  VectorParamsAs1DForOutWhenUnconnected=off
  wires:
  AccelIn/1 -> Accel/1
  DecelIn/1 -> Decel/1
  Constant/1 -> Gear/1
  Constant1/1 -> Clutch/1
  VehFdbk/1 -> Terminator1/1
  ExtGear/1 -> Terminator2/1
  VehRef/1 -> Terminator3/1

== system Driver_Long_Lat_Stanley/Long Lat Stanley/Longitudinal Driver/Longitudinal Driver/Shift/Scheduled ==
  AccelIn : Inport
  DecelIn : Inport  Port=2
  VehRef : Inport  Port=3
  VehFdbk : Inport  Port=4
  ExtGear : Inport  Port=5
  Reverse Change : autolibsharedcommon/Longitudinal Driver/Shift/Basic/Reverse Change  SystemSampleTime=-1  VariantActivationTime=update diagram  Latency=0  AutoFrameSizeCalculation=off
      settings: SourceProductBaseCode=PW,MT,UV,VE,VP
  Shift Controller : Stateflow chart  TreatAsAtomicUnit=on
  Terminator : Terminator
  Accel : Outport  VectorParamsAs1DForOutWhenUnconnected=off
  Decel : Outport  Port=2  VectorParamsAs1DForOutWhenUnconnected=off
  Gear : Outport  Port=3  VectorParamsAs1DForOutWhenUnconnected=off
  Clutch : Outport  Port=4  VectorParamsAs1DForOutWhenUnconnected=off
  wires:
  Shift Controller/1(Gear) -> Gear/1, Reverse Change/3
  AccelIn/1 -> Shift Controller/1(pedal), Reverse Change/1
  VehFdbk/1 -> Shift Controller/4(speed)
  VehRef/1 -> [VehRef], Shift Controller/3(VehRef)
  DecelIn/1 -> Reverse Change/2, Shift Controller/2(Brake)
  Shift Controller/2(clutchControl) -> Clutch/1
  Reverse Change/1 -> Accel/1
  Reverse Change/2 -> Decel/1
  ExtGear/1 -> Terminator/1
  [VehRef] -> Reverse Change/4

== system Driver_Long_Lat_Stanley/Long Lat Stanley/Longitudinal Driver/Longitudinal Driver/Control/Mapped/Accel Override ==
  u_o(t) : Inport
  ExtActions : Inport  Port=2
  0~1 : Saturate  UpperLimit=1  LowerLimit=0  ZeroCross=off
  Bus Selector1 : BusSelector  OutputSignals=AccelHld,EnblAccelOvr,AccelOvrCmd,AccelZero
  Constant : Constant  Value=0
  Enabled Subsystem : Subsystem  TreatAsAtomicUnit=on
  Logical Operator1 : Logic  Operator=NOT  AllPortsSameDT=off  OutDataTypeStr=boolean
  Logical Operator2 : Logic  AllPortsSameDT=off  OutDataTypeStr=boolean
  Logical Operator3 : Logic  AllPortsSameDT=off  OutDataTypeStr=boolean
  NOT : Logic  Operator=NOT  IconShape=distinctive  AllPortsSameDT=off  OutDataTypeStr=boolean
  Saturation1 : Saturate  UpperLimit=1  LowerLimit=0  ZeroCross=off
  Switch : Switch  Criteria=u2 > Threshold
  Switch1 : Switch  Criteria=u2 > Threshold
  u : Outport
  Accel : Outport  Port=2
  wires:
  Logical Operator3/1 -> NOT/1
  u_o(t)/1 -> 0~1/1
  0~1/1 -> Switch/3  "Accel"
  Bus Selector1/1 -> Logical Operator3/1  "<AccelHld>"
  Bus Selector1/3 -> Switch1/1  "<AccelOvrCmd>"
  Bus Selector1/2 -> Logical Operator2/1  "<EnblAccelOvr>"
  Bus Selector1/4 -> Switch/2, Logical Operator1/1  "<AccelZero>"
  Logical Operator1/1 -> Logical Operator2/2, Logical Operator3/2
  Logical Operator2/1 -> Switch1/2
  Saturation1/1 -> u/1, Accel/1
  Switch1/1 -> Enabled Subsystem/1(In1)
  Constant/1 -> Switch/1
  ExtActions/1 -> Bus Selector1/1
  Switch/1 -> Switch1/3  "u(t)"
  NOT/1 -> Enabled Subsystem/Enable
  Enabled Subsystem/1(Out1) -> Saturation1/1

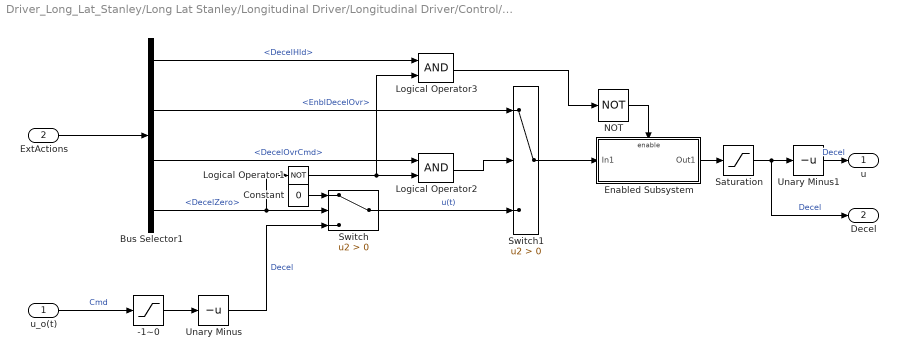
== system Driver_Long_Lat_Stanley/Long Lat Stanley/Longitudinal Driver/Longitudinal Driver/Control/Mapped/Deccel Override ==
  u_o(t) : Inport
  ExtActions : Inport  Port=2
  -1~0 : Saturate  UpperLimit=0  LowerLimit=-1  ZeroCross=off
  Bus Selector1 : BusSelector  OutputSignals=DecelHld,EnblDecelOvr,DecelOvrCmd,DecelZero
  Constant : Constant  Value=0
  Enabled Subsystem : Subsystem  TreatAsAtomicUnit=on
  Logical Operator1 : Logic  Operator=NOT  AllPortsSameDT=off  OutDataTypeStr=boolean
  Logical Operator2 : Logic  AllPortsSameDT=off  OutDataTypeStr=boolean
  Logical Operator3 : Logic  AllPortsSameDT=off  OutDataTypeStr=boolean
  NOT : Logic  Operator=NOT  IconShape=distinctive  AllPortsSameDT=off  OutDataTypeStr=boolean
  Saturation : Saturate  UpperLimit=1  LowerLimit=0  ZeroCross=off
  Switch : Switch  Criteria=u2 > Threshold
  Switch1 : Switch  Criteria=u2 > Threshold
  Unary Minus : UnaryMinus
  Unary Minus1 : UnaryMinus
  u : Outport
  Decel : Outport  Port=2
  wires:
  Unary Minus1/1 -> u/1  "Decel"
  Saturation/1 -> Decel/1, Unary Minus1/1  "Decel"
  Unary Minus/1 -> Switch/3  "Decel"
  u_o(t)/1 -> -1~0/1  "Cmd"
  -1~0/1 -> Unary Minus/1
  Switch/1 -> Switch1/3  "u(t)"
  ExtActions/1 -> Bus Selector1/1
  Constant/1 -> Switch/1
  Enabled Subsystem/1(Out1) -> Saturation/1
  Switch1/1 -> Enabled Subsystem/1(In1)
  Logical Operator3/1 -> NOT/1
  Logical Operator2/1 -> Switch1/2
  Logical Operator1/1 -> Logical Operator3/2, Logical Operator2/2
  Bus Selector1/4 -> Logical Operator1/1, Switch/2  "<DecelZero>"
  Bus Selector1/1 -> Logical Operator3/1  "<DecelHld>"
  Bus Selector1/2 -> Switch1/1  "<EnblDecelOvr>"
  Bus Selector1/3 -> Logical Operator2/1  "<DecelOvrCmd>"
  NOT/1 -> Enabled Subsystem/Enable

== system Driver_Long_Lat_Stanley/Long Lat Stanley/Longitudinal Driver/Longitudinal Driver/Control/Predictive/Accel Override ==
  u_o(t) : Inport
  ExtActions : Inport  Port=2
  0~1 : Saturate  UpperLimit=1  LowerLimit=0  ZeroCross=off
  Bus Selector1 : BusSelector  OutputSignals=AccelHld,EnblAccelOvr,AccelOvrCmd,AccelZero
  Constant : Constant  Value=0
  Enabled Subsystem : Subsystem  TreatAsAtomicUnit=on
  Logical Operator1 : Logic  Operator=NOT  AllPortsSameDT=off  OutDataTypeStr=boolean
  Logical Operator2 : Logic  AllPortsSameDT=off  OutDataTypeStr=boolean
  Logical Operator3 : Logic  AllPortsSameDT=off  OutDataTypeStr=boolean
  NOT : Logic  Operator=NOT  IconShape=distinctive  AllPortsSameDT=off  OutDataTypeStr=boolean
  Saturation1 : Saturate  UpperLimit=1  LowerLimit=0  ZeroCross=off
  Switch : Switch  Criteria=u2 > Threshold
  Switch1 : Switch  Criteria=u2 > Threshold
  u : Outport
  Accel : Outport  Port=2
  wires:
  Logical Operator3/1 -> NOT/1
  u_o(t)/1 -> 0~1/1
  0~1/1 -> Switch/3  "Accel"
  Bus Selector1/1 -> Logical Operator3/1  "<AccelHld>"
  Bus Selector1/3 -> Switch1/1  "<AccelOvrCmd>"
  Bus Selector1/2 -> Logical Operator2/1  "<EnblAccelOvr>"
  Bus Selector1/4 -> Switch/2, Logical Operator1/1  "<AccelZero>"
  Logical Operator1/1 -> Logical Operator2/2, Logical Operator3/2
  Logical Operator2/1 -> Switch1/2
  Saturation1/1 -> u/1, Accel/1
  Switch1/1 -> Enabled Subsystem/1(In1)
  Constant/1 -> Switch/1
  ExtActions/1 -> Bus Selector1/1
  Switch/1 -> Switch1/3  "u(t)"
  NOT/1 -> Enabled Subsystem/Enable
  Enabled Subsystem/1(Out1) -> Saturation1/1

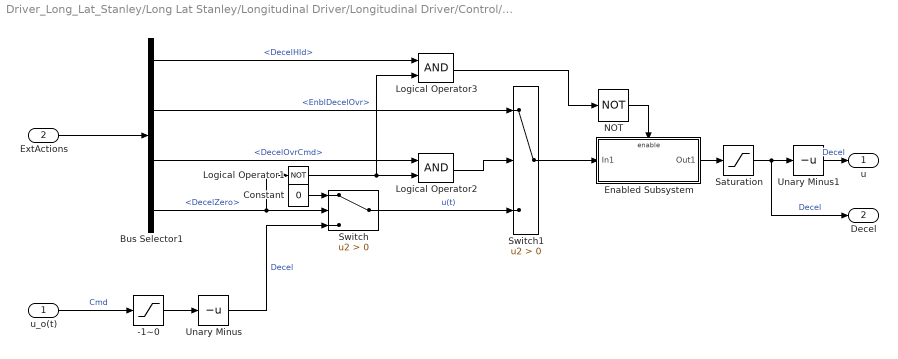
== system Driver_Long_Lat_Stanley/Long Lat Stanley/Longitudinal Driver/Longitudinal Driver/Control/Predictive/Deccel Override ==
  u_o(t) : Inport
  ExtActions : Inport  Port=2
  -1~0 : Saturate  UpperLimit=0  LowerLimit=-1  ZeroCross=off
  Bus Selector1 : BusSelector  OutputSignals=DecelHld,EnblDecelOvr,DecelOvrCmd,DecelZero
  Constant : Constant  Value=0
  Enabled Subsystem : Subsystem  TreatAsAtomicUnit=on
  Logical Operator1 : Logic  Operator=NOT  AllPortsSameDT=off  OutDataTypeStr=boolean
  Logical Operator2 : Logic  AllPortsSameDT=off  OutDataTypeStr=boolean
  Logical Operator3 : Logic  AllPortsSameDT=off  OutDataTypeStr=boolean
  NOT : Logic  Operator=NOT  IconShape=distinctive  AllPortsSameDT=off  OutDataTypeStr=boolean
  Saturation : Saturate  UpperLimit=1  LowerLimit=0  ZeroCross=off
  Switch : Switch  Criteria=u2 > Threshold
  Switch1 : Switch  Criteria=u2 > Threshold
  Unary Minus : UnaryMinus
  Unary Minus1 : UnaryMinus
  u : Outport
  Decel : Outport  Port=2
  wires:
  Unary Minus1/1 -> u/1  "Decel"
  Saturation/1 -> Decel/1, Unary Minus1/1  "Decel"
  Unary Minus/1 -> Switch/3  "Decel"
  u_o(t)/1 -> -1~0/1  "Cmd"
  -1~0/1 -> Unary Minus/1
  Switch/1 -> Switch1/3  "u(t)"
  ExtActions/1 -> Bus Selector1/1
  Constant/1 -> Switch/1
  Enabled Subsystem/1(Out1) -> Saturation/1
  Switch1/1 -> Enabled Subsystem/1(In1)
  Logical Operator3/1 -> NOT/1
  Logical Operator2/1 -> Switch1/2
  Logical Operator1/1 -> Logical Operator3/2, Logical Operator2/2
  Bus Selector1/4 -> Logical Operator1/1, Switch/2  "<DecelZero>"
  Bus Selector1/1 -> Logical Operator3/1  "<DecelHld>"
  Bus Selector1/2 -> Switch1/1  "<EnblDecelOvr>"
  Bus Selector1/3 -> Logical Operator2/1  "<DecelOvrCmd>"
  NOT/1 -> Enabled Subsystem/Enable

== system Driver_Long_Lat_Stanley/Long Lat Stanley/Longitudinal Driver/Longitudinal Driver/Control/Predictive/Powertrain Response ==
  "u " : Inport
  Filtered : Subsystem  VariantControl=1
  Unfiltered : Subsystem  VariantControl=0
  " u'" : Outport  VectorParamsAs1DForOutWhenUnconnected=off

== system Driver_Long_Lat_Stanley/Long Lat Stanley/Longitudinal Driver/Longitudinal Driver/Control/Scalar/Accel Override ==
  u_o(t) : Inport
  ExtActions : Inport  Port=2
  0~1 : Saturate  UpperLimit=1  LowerLimit=0  ZeroCross=off
  Bus Selector1 : BusSelector  OutputSignals=AccelHld,EnblAccelOvr,AccelOvrCmd,AccelZero
  Constant : Constant  Value=0
  Enabled Subsystem : Subsystem  TreatAsAtomicUnit=on
  Logical Operator1 : Logic  Operator=NOT  AllPortsSameDT=off  OutDataTypeStr=boolean
  Logical Operator2 : Logic  AllPortsSameDT=off  OutDataTypeStr=boolean
  Logical Operator3 : Logic  AllPortsSameDT=off  OutDataTypeStr=boolean
  NOT : Logic  Operator=NOT  IconShape=distinctive  AllPortsSameDT=off  OutDataTypeStr=boolean
  Saturation1 : Saturate  UpperLimit=1  LowerLimit=0  ZeroCross=off
  Switch : Switch  Criteria=u2 > Threshold
  Switch1 : Switch  Criteria=u2 > Threshold
  u : Outport
  Accel : Outport  Port=2
  wires:
  Logical Operator3/1 -> NOT/1
  u_o(t)/1 -> 0~1/1
  0~1/1 -> Switch/3  "Accel"
  Bus Selector1/1 -> Logical Operator3/1  "<AccelHld>"
  Bus Selector1/3 -> Switch1/1  "<AccelOvrCmd>"
  Bus Selector1/2 -> Logical Operator2/1  "<EnblAccelOvr>"
  Bus Selector1/4 -> Switch/2, Logical Operator1/1  "<AccelZero>"
  Logical Operator1/1 -> Logical Operator2/2, Logical Operator3/2
  Logical Operator2/1 -> Switch1/2
  Saturation1/1 -> u/1, Accel/1
  Switch1/1 -> Enabled Subsystem/1(In1)
  Constant/1 -> Switch/1
  ExtActions/1 -> Bus Selector1/1
  Switch/1 -> Switch1/3  "u(t)"
  NOT/1 -> Enabled Subsystem/Enable
  Enabled Subsystem/1(Out1) -> Saturation1/1

== system Driver_Long_Lat_Stanley/Long Lat Stanley/Longitudinal Driver/Longitudinal Driver/Control/Scalar/Deccel Override ==
  u_o(t) : Inport
  ExtActions : Inport  Port=2
  -1~0 : Saturate  UpperLimit=0  LowerLimit=-1  ZeroCross=off
  Bus Selector1 : BusSelector  OutputSignals=DecelHld,EnblDecelOvr,DecelOvrCmd,DecelZero
  Constant : Constant  Value=0
  Enabled Subsystem : Subsystem  TreatAsAtomicUnit=on
  Logical Operator1 : Logic  Operator=NOT  AllPortsSameDT=off  OutDataTypeStr=boolean
  Logical Operator2 : Logic  AllPortsSameDT=off  OutDataTypeStr=boolean
  Logical Operator3 : Logic  AllPortsSameDT=off  OutDataTypeStr=boolean
  NOT : Logic  Operator=NOT  IconShape=distinctive  AllPortsSameDT=off  OutDataTypeStr=boolean
  Saturation : Saturate  UpperLimit=1  LowerLimit=0  ZeroCross=off
  Switch : Switch  Criteria=u2 > Threshold
  Switch1 : Switch  Criteria=u2 > Threshold
  Unary Minus : UnaryMinus
  Unary Minus1 : UnaryMinus
  u : Outport
  Decel : Outport  Port=2
  wires:
  Unary Minus1/1 -> u/1  "Decel"
  Saturation/1 -> Decel/1, Unary Minus1/1  "Decel"
  Unary Minus/1 -> Switch/3  "Decel"
  u_o(t)/1 -> -1~0/1  "Cmd"
  -1~0/1 -> Unary Minus/1
  Switch/1 -> Switch1/3  "u(t)"
  ExtActions/1 -> Bus Selector1/1
  Constant/1 -> Switch/1
  Enabled Subsystem/1(Out1) -> Saturation/1
  Switch1/1 -> Enabled Subsystem/1(In1)
  Logical Operator3/1 -> NOT/1
  Logical Operator2/1 -> Switch1/2
  Logical Operator1/1 -> Logical Operator3/2, Logical Operator2/2
  Bus Selector1/4 -> Logical Operator1/1, Switch/2  "<DecelZero>"
  Bus Selector1/1 -> Logical Operator3/1  "<DecelHld>"
  Bus Selector1/2 -> Switch1/1  "<EnblDecelOvr>"
  Bus Selector1/3 -> Logical Operator2/1  "<DecelOvrCmd>"
  NOT/1 -> Enabled Subsystem/Enable
